simulink subsystem "airCoolingDuty"  (R2022b)
settings: Solver=VariableStepAuto  StartTime=0.0  StopTime=10.0  RelTol=1e-3
libraries: cooling_lib x8, Raptor_lib x8
settings Model: Creator=serga  LastModifiedBy=serga

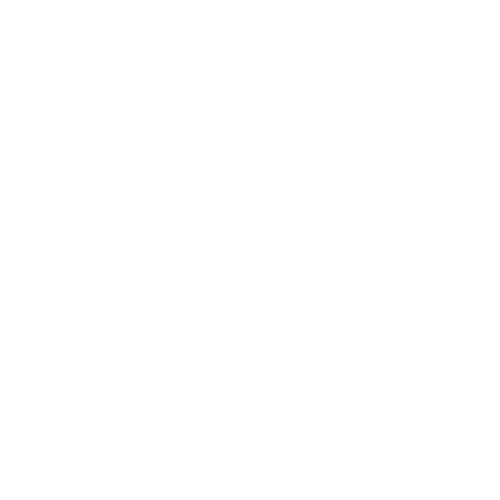
[thumbnail: Simulink's stored preview of the top-level diagram]
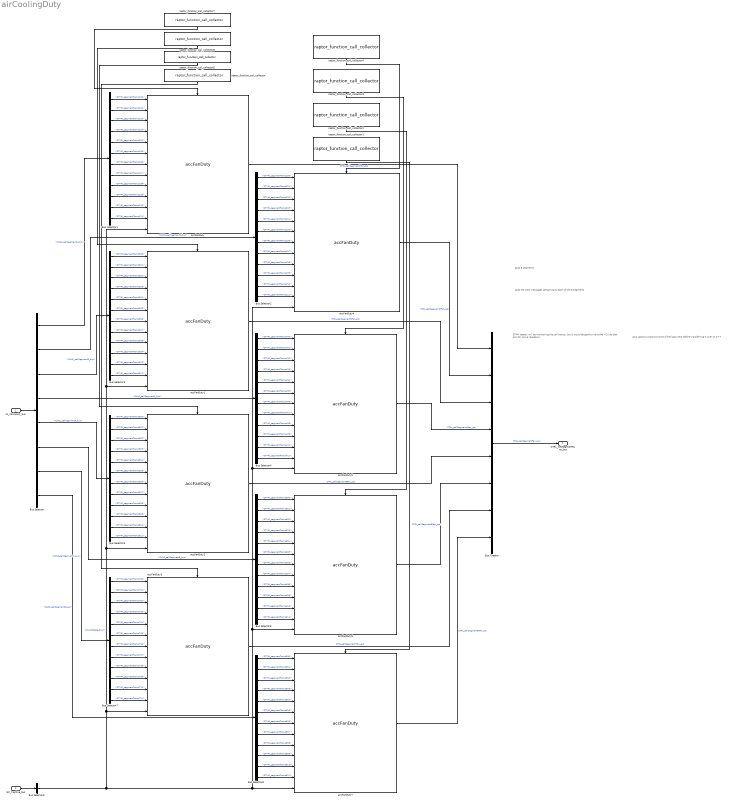
== system airCoolingDuty ==
  note: also, good to practice some of the logic here before transferring it over to C++
  note: STMM teensy will be monitoring the cell temps, but it would be good to have the VCU do that also for some redudancy
  note: grab the CAN messages pertaining to each of the 8 segments
  note: grab 8 segments
  IN_canInputs_bus : Inport
  SM_tractive_bus : Inport  Port=2
  Bus Creator : BusCreator  Inputs=8
  Bus Selector : BusSelector  OutputSignals=IN_can2Inputs_bus.CAN2_stmm_bus.CAN2_cellSegment1_bus,IN_can2Inputs_bus.CAN2_stmm_bus.CAN2_cellSegment2_bus,IN_can2Inputs_bus.CAN2_stmm_bus.CAN2_cellSegment3_bus,IN_can2Inputs_bus.CAN2_stmm_bus.CAN2_cellSegment4_bus,IN_can2Inputs_bus.CAN2_stmm_bus.CAN2_cellSegment5_bus,IN_can2Inputs_bus.CAN2_stmm_bus.CAN2_cellSegment6_bus,IN_can2Inputs_bus.CAN2_stmm_bus.CAN2_cellSegment7_bus,IN_can2Inputs_bus.CAN2_stmm_bus.CAN2_cellSegment8_bus
  Bus Selector1 : BusSelector  OutputSignals=CAN2_stmm_300_bus.STMM_segmentTemp100,CAN2_stmm_300_bus.STMM_segmentTemp101,CAN2_stmm_300_bus.STMM_segmentTemp102,CAN2_stmm_301_bus.STMM_segmentTemp103,CAN2_stmm_301_bus.STMM_segmentTemp104,CAN2_stmm_301_bus.STMM_segmentTemp105,CAN2_stmm_302_bus.STMM_segmentTemp106,CAN2_stmm_302_bus.STMM_segmentTemp107,CAN2_stmm_302_bus.STMM_segmentTemp108,CAN2_stmm_303_bus.STMM_segmentTemp109,CAN2_stmm_303_bus.STMM_segmentTemp110,CAN2_stmm_303_bus.STMM_segmentTemp111
  Bus Selector2 : BusSelector  OutputSignals=CAN2_stmm_304_bus.STMM_segmentTemp200,CAN2_stmm_304_bus.STMM_segmentTemp201,CAN2_stmm_304_bus.STMM_segmentTemp202,CAN2_stmm_305_bus.STMM_segmentTemp203,CAN2_stmm_305_bus.STMM_segmentTemp204,CAN2_stmm_305_bus.STMM_segmentTemp205,CAN2_stmm_306_bus.STMM_segmentTemp206,CAN2_stmm_306_bus.STMM_segmentTemp207,CAN2_stmm_306_bus.STMM_segmentTemp208,CAN2_stmm_307_bus.STMM_segmentTemp209,CAN2_stmm_307_bus.STMM_segmentTemp210,CAN2_stmm_307_bus.STMM_segmentTemp211
  Bus Selector3 : BusSelector  OutputSignals=CAN2_stmm_308_bus.STMM_segmentTemp300,CAN2_stmm_308_bus.STMM_segmentTemp301,CAN2_stmm_308_bus.STMM_segmentTemp302,CAN2_stmm_309_bus.STMM_segmentTemp303,CAN2_stmm_309_bus.STMM_segmentTemp304,CAN2_stmm_309_bus.STMM_segmentTemp305,CAN2_stmm_310_bus.STMM_segmentTemp306,CAN2_stmm_310_bus.STMM_segmentTemp307,CAN2_stmm_310_bus.STMM_segmentTemp308,CAN2_stmm_311_bus.STMM_segmentTemp309,CAN2_stmm_311_bus.STMM_segmentTemp310,CAN2_stmm_311_bus.STMM_segmentTemp311
  Bus Selector4 : BusSelector  OutputSignals=CAN2_stmm_312_bus.STMM_segmentTemp400,CAN2_stmm_312_bus.STMM_segmentTemp401,CAN2_stmm_312_bus.STMM_segmentTemp402,CAN2_stmm_313_bus.STMM_segmentTemp403,CAN2_stmm_313_bus.STMM_segmentTemp404,CAN2_stmm_313_bus.STMM_segmentTemp405,CAN2_stmm_314_bus.STMM_segmentTemp406,CAN2_stmm_314_bus.STMM_segmentTemp407,CAN2_stmm_314_bus.STMM_segmentTemp408,CAN2_stmm_315_bus.STMM_segmentTemp409,CAN2_stmm_315_bus.STMM_segmentTemp410,CAN2_stmm_315_bus.STMM_segmentTemp411
  Bus Selector5 : BusSelector  OutputSignals=CAN2_stmm_316_bus.STMM_segmentTemp500,CAN2_stmm_316_bus.STMM_segmentTemp501,CAN2_stmm_316_bus.STMM_segmentTemp502,CAN2_stmm_317_bus.STMM_segmentTemp503,CAN2_stmm_317_bus.STMM_segmentTemp504,CAN2_stmm_317_bus.STMM_segmentTemp505,CAN2_stmm_318_bus.STMM_segmentTemp506,CAN2_stmm_318_bus.STMM_segmentTemp507,CAN2_stmm_318_bus.STMM_segmentTemp508,CAN2_stmm_319_bus.STMM_segmentTemp509,CAN2_stmm_319_bus.STMM_segmentTemp510,CAN2_stmm_319_bus.STMM_segmentTemp511
  Bus Selector6 : BusSelector  OutputSignals=CAN2_stmm_320_bus.STMM_segmentTemp600,CAN2_stmm_320_bus.STMM_segmentTemp601,CAN2_stmm_320_bus.STMM_segmentTemp602,CAN2_stmm_321_bus.STMM_segmentTemp603,CAN2_stmm_321_bus.STMM_segmentTemp604,CAN2_stmm_321_bus.STMM_segmentTemp605,CAN2_stmm_322_bus.STMM_segmentTemp606,CAN2_stmm_322_bus.STMM_segmentTemp607,CAN2_stmm_322_bus.STMM_segmentTemp608,CAN2_stmm_323_bus.STMM_segmentTemp609,CAN2_stmm_323_bus.STMM_segmentTemp610,CAN2_stmm_323_bus.STMM_segmentTemp611
  Bus Selector7 : BusSelector  OutputSignals=CAN2_stmm_324_bus.STMM_segmentTemp700,CAN2_stmm_324_bus.STMM_segmentTemp701,CAN2_stmm_324_bus.STMM_segmentTemp702,CAN2_stmm_325_bus.STMM_segmentTemp703,CAN2_stmm_325_bus.STMM_segmentTemp704,CAN2_stmm_325_bus.STMM_segmentTemp705,CAN2_stmm_326_bus.STMM_segmentTemp706,CAN2_stmm_326_bus.STMM_segmentTemp707,CAN2_stmm_326_bus.STMM_segmentTemp708,CAN2_stmm_327_bus.STMM_segmentTemp709,CAN2_stmm_327_bus.STMM_segmentTemp710,CAN2_stmm_327_bus.STMM_segmentTemp711
  Bus Selector8 : BusSelector  OutputSignals=CAN2_stmm_328_bus.STMM_segmentTemp800,CAN2_stmm_328_bus.STMM_segmentTemp801,CAN2_stmm_328_bus.STMM_segmentTemp802,CAN2_stmm_329_bus.STMM_segmentTemp803,CAN2_stmm_329_bus.STMM_segmentTemp804,CAN2_stmm_329_bus.STMM_segmentTemp805,CAN2_stmm_330_bus.STMM_segmentTemp806,CAN2_stmm_330_bus.STMM_segmentTemp807,CAN2_stmm_330_bus.STMM_segmentTemp808,CAN2_stmm_331_bus.STMM_segmentTemp809,CAN2_stmm_331_bus.STMM_segmentTemp810,CAN2_stmm_331_bus.STMM_segmentTemp811
  Bus Selector9 : BusSelector  OutputSignals=SM_rtdState_bool
  accFanDuty : cooling_lib/accFanDuty  pos='1'
  accFanDuty1 : cooling_lib/accFanDuty  pos='3'
  accFanDuty2 : cooling_lib/accFanDuty  pos='5'
  accFanDuty3 : cooling_lib/accFanDuty  pos='7'
  accFanDuty4 : cooling_lib/accFanDuty  pos='2'
  accFanDuty5 : cooling_lib/accFanDuty  pos='4'
  accFanDuty6 : cooling_lib/accFanDuty  pos='6'
  accFanDuty7 : cooling_lib/accFanDuty  pos='8'
  raptor_function_call_collector{,1..7} (8 alike) : Raptor_lib/Triggers/raptor_function_call_collector  count=5
      settings: SourceProductName=Raptor
  CTRL_cellSegmentFans_bus : Outport
  wires:
  raptor_function_call_collector/1 -> accFanDuty3/Trigger
  raptor_function_call_collector5/1 -> accFanDuty2/Trigger
  raptor_function_call_collector6/1 -> accFanDuty1/Trigger
  raptor_function_call_collector7/1 -> accFanDuty/Trigger
  raptor_function_call_collector1/1 -> accFanDuty7/Trigger
  raptor_function_call_collector2/1 -> accFanDuty6/Trigger
  raptor_function_call_collector3/1 -> accFanDuty5/Trigger
  raptor_function_call_collector4/1 -> accFanDuty4/Trigger
  Bus Creator/1 -> CTRL_cellSegmentFans_bus/1  "CTRL_cellSegmentFan_bus"
  Bus Selector9/1 -> accFanDuty4/13, accFanDuty5/13, accFanDuty6/13, accFanDuty7/13, accFanDuty1/13, accFanDuty/13, accFanDuty2/13, accFanDuty3/13  "<SM_rtdState_bool>"
  IN_canInputs_bus/1 -> Bus Selector/1
  Bus Selector/1 -> Bus Selector1/1  "<CAN2_cellSegment1_bus>"
  Bus Selector/2 -> Bus Selector2/1  "<CAN2_cellSegment2_bus>"
  Bus Selector/3 -> Bus Selector3/1  "<CAN2_cellSegment3_bus>"
  Bus Selector/4 -> Bus Selector4/1  "<CAN2_cellSegment4_bus>"
  Bus Selector/5 -> Bus Selector5/1  "<CAN2_cellSegment5_bus>"
  Bus Selector/6 -> Bus Selector6/1  "<CAN2_cellSegment6_bus>"
  Bus Selector/7 -> Bus Selector7/1  "<CAN2_cellSegment7_bus>"
  Bus Selector/8 -> Bus Selector8/1  "<CAN2_cellSegment8_bus>"
  Bus Selector1/1 -> accFanDuty/1  "<STMM_segmentTemp100>"
  Bus Selector1/3 -> accFanDuty/3  "<STMM_segmentTemp102>"
  Bus Selector1/2 -> accFanDuty/2  "<STMM_segmentTemp101>"
  Bus Selector1/4 -> accFanDuty/4  "<STMM_segmentTemp103>"
  Bus Selector1/5 -> accFanDuty/5  "<STMM_segmentTemp104>"
  Bus Selector1/6 -> accFanDuty/6  "<STMM_segmentTemp105>"
  Bus Selector1/7 -> accFanDuty/7  "<STMM_segmentTemp106>"
  Bus Selector1/8 -> accFanDuty/8  "<STMM_segmentTemp107>"
  Bus Selector1/9 -> accFanDuty/9  "<STMM_segmentTemp108>"
  Bus Selector1/10 -> accFanDuty/10  "<STMM_segmentTemp109>"
  Bus Selector1/11 -> accFanDuty/11  "<STMM_segmentTemp110>"
  Bus Selector1/12 -> accFanDuty/12  "<STMM_segmentTemp111>"
  Bus Selector3/7 -> accFanDuty1/7  "<STMM_segmentTemp306>"
  Bus Selector3/6 -> accFanDuty1/6  "<STMM_segmentTemp305>"
  Bus Selector3/5 -> accFanDuty1/5  "<STMM_segmentTemp304>"
  Bus Selector3/4 -> accFanDuty1/4  "<STMM_segmentTemp303>"
  Bus Selector3/3 -> accFanDuty1/3  "<STMM_segmentTemp302>"
  Bus Selector3/8 -> accFanDuty1/8  "<STMM_segmentTemp307>"
  Bus Selector3/9 -> accFanDuty1/9  "<STMM_segmentTemp308>"
  Bus Selector3/10 -> accFanDuty1/10  "<STMM_segmentTemp309>"
  Bus Selector3/11 -> accFanDuty1/11  "<STMM_segmentTemp310>"
  Bus Selector3/12 -> accFanDuty1/12  "<STMM_segmentTemp311>"
  Bus Selector3/2 -> accFanDuty1/2  "<STMM_segmentTemp301>"
  Bus Selector3/1 -> accFanDuty1/1  "<STMM_segmentTemp300>"
  Bus Selector5/1 -> accFanDuty2/1  "<STMM_segmentTemp500>"
  Bus Selector5/2 -> accFanDuty2/2  "<STMM_segmentTemp501>"
  Bus Selector5/3 -> accFanDuty2/3  "<STMM_segmentTemp502>"
  Bus Selector5/4 -> accFanDuty2/4  "<STMM_segmentTemp503>"
  Bus Selector5/5 -> accFanDuty2/5  "<STMM_segmentTemp504>"
  Bus Selector5/6 -> accFanDuty2/6  "<STMM_segmentTemp505>"
  Bus Selector5/7 -> accFanDuty2/7  "<STMM_segmentTemp506>"
  Bus Selector5/8 -> accFanDuty2/8  "<STMM_segmentTemp507>"
  Bus Selector5/9 -> accFanDuty2/9  "<STMM_segmentTemp508>"
  Bus Selector5/10 -> accFanDuty2/10  "<STMM_segmentTemp509>"
  Bus Selector5/11 -> accFanDuty2/11  "<STMM_segmentTemp510>"
  Bus Selector5/12 -> accFanDuty2/12  "<STMM_segmentTemp511>"
  Bus Selector7/6 -> accFanDuty3/6  "<STMM_segmentTemp705>"
  Bus Selector7/1 -> accFanDuty3/1  "<STMM_segmentTemp700>"
  Bus Selector7/2 -> accFanDuty3/2  "<STMM_segmentTemp701>"
  Bus Selector7/3 -> accFanDuty3/3  "<STMM_segmentTemp702>"
  Bus Selector7/4 -> accFanDuty3/4  "<STMM_segmentTemp703>"
  Bus Selector7/5 -> accFanDuty3/5  "<STMM_segmentTemp704>"
  Bus Selector7/7 -> accFanDuty3/7  "<STMM_segmentTemp706>"
  Bus Selector7/8 -> accFanDuty3/8  "<STMM_segmentTemp707>"
  Bus Selector7/9 -> accFanDuty3/9  "<STMM_segmentTemp708>"
  Bus Selector7/10 -> accFanDuty3/10  "<STMM_segmentTemp709>"
  Bus Selector7/11 -> accFanDuty3/11  "<STMM_segmentTemp710>"
  Bus Selector7/12 -> accFanDuty3/12  "<STMM_segmentTemp711>"
  Bus Selector2/1 -> accFanDuty4/1  "<STMM_segmentTemp200>"
  Bus Selector2/2 -> accFanDuty4/2  "<STMM_segmentTemp201>"
  Bus Selector2/3 -> accFanDuty4/3  "<STMM_segmentTemp202>"
  Bus Selector2/4 -> accFanDuty4/4  "<STMM_segmentTemp203>"
  Bus Selector2/5 -> accFanDuty4/5  "<STMM_segmentTemp204>"
  Bus Selector2/6 -> accFanDuty4/6  "<STMM_segmentTemp205>"
  Bus Selector2/7 -> accFanDuty4/7  "<STMM_segmentTemp206>"
  Bus Selector2/8 -> accFanDuty4/8  "<STMM_segmentTemp207>"
  Bus Selector2/9 -> accFanDuty4/9  "<STMM_segmentTemp208>"
  Bus Selector2/10 -> accFanDuty4/10  "<STMM_segmentTemp209>"
  Bus Selector2/11 -> accFanDuty4/11  "<STMM_segmentTemp210>"
  Bus Selector2/12 -> accFanDuty4/12  "<STMM_segmentTemp211>"
  Bus Selector4/1 -> accFanDuty5/1  "<STMM_segmentTemp400>"
  Bus Selector4/2 -> accFanDuty5/2  "<STMM_segmentTemp401>"
  Bus Selector4/3 -> accFanDuty5/3  "<STMM_segmentTemp402>"
  Bus Selector4/4 -> accFanDuty5/4  "<STMM_segmentTemp403>"
  Bus Selector4/5 -> accFanDuty5/5  "<STMM_segmentTemp404>"
  Bus Selector4/6 -> accFanDuty5/6  "<STMM_segmentTemp405>"
  Bus Selector4/8 -> accFanDuty5/8  "<STMM_segmentTemp407>"
  Bus Selector4/7 -> accFanDuty5/7  "<STMM_segmentTemp406>"
  Bus Selector4/9 -> accFanDuty5/9  "<STMM_segmentTemp408>"
  Bus Selector4/11 -> accFanDuty5/11  "<STMM_segmentTemp410>"
  Bus Selector4/10 -> accFanDuty5/10  "<STMM_segmentTemp409>"
  Bus Selector4/12 -> accFanDuty5/12  "<STMM_segmentTemp411>"
  Bus Selector6/1 -> accFanDuty6/1  "<STMM_segmentTemp600>"
  Bus Selector6/2 -> accFanDuty6/2  "<STMM_segmentTemp601>"
  Bus Selector6/3 -> accFanDuty6/3  "<STMM_segmentTemp602>"
  Bus Selector6/4 -> accFanDuty6/4  "<STMM_segmentTemp603>"
  Bus Selector6/5 -> accFanDuty6/5  "<STMM_segmentTemp604>"
  Bus Selector6/6 -> accFanDuty6/6  "<STMM_segmentTemp605>"
  Bus Selector6/7 -> accFanDuty6/7  "<STMM_segmentTemp606>"
  Bus Selector6/8 -> accFanDuty6/8  "<STMM_segmentTemp607>"
  Bus Selector6/9 -> accFanDuty6/9  "<STMM_segmentTemp608>"
  Bus Selector6/10 -> accFanDuty6/10  "<STMM_segmentTemp609>"
  Bus Selector6/11 -> accFanDuty6/11  "<STMM_segmentTemp610>"
  Bus Selector6/12 -> accFanDuty6/12  "<STMM_segmentTemp611>"
  Bus Selector8/1 -> accFanDuty7/1  "<STMM_segmentTemp800>"
  Bus Selector8/2 -> accFanDuty7/2  "<STMM_segmentTemp801>"
  Bus Selector8/3 -> accFanDuty7/3  "<STMM_segmentTemp802>"
  Bus Selector8/4 -> accFanDuty7/4  "<STMM_segmentTemp803>"
  Bus Selector8/5 -> accFanDuty7/5  "<STMM_segmentTemp804>"
  Bus Selector8/6 -> accFanDuty7/6  "<STMM_segmentTemp805>"
  Bus Selector8/7 -> accFanDuty7/7  "<STMM_segmentTemp806>"
  Bus Selector8/8 -> accFanDuty7/8  "<STMM_segmentTemp807>"
  Bus Selector8/9 -> accFanDuty7/9  "<STMM_segmentTemp808>"
  Bus Selector8/10 -> accFanDuty7/10  "<STMM_segmentTemp809>"
  Bus Selector8/11 -> accFanDuty7/11  "<STMM_segmentTemp810>"
  Bus Selector8/12 -> accFanDuty7/12  "<STMM_segmentTemp811>"
  accFanDuty/1 -> Bus Creator/1  "CTRL_cellSegment1Fan_pct"
  accFanDuty4/1 -> Bus Creator/2  "CTRL_cellSegment2Fan_pct"
  accFanDuty1/1 -> Bus Creator/3  "CTRL_cellSegment3Fan_pct"
  accFanDuty5/1 -> Bus Creator/4  "CTRL_cellSegment4Fan_pct"
  accFanDuty2/1 -> Bus Creator/5  "CTRL_cellSegment5Fan_pct"
  accFanDuty6/1 -> Bus Creator/6  "CTRL_cellSegment6Fan_pct"
  accFanDuty3/1 -> Bus Creator/7  "CTRL_cellSegment7Fan_pct"
  accFanDuty7/1 -> Bus Creator/8  "CTRL_cellSegment8Fan_pct"
  SM_tractive_bus/1 -> Bus Selector9/1
